simulink model "Lab3_12082026"  (R2019a)
settings: Solver=VariableStepAuto  StartTime=0.0  StopTime=10  RelTol=1e-3  EnableMultiTasking=on
libraries: dspsrcs4 x1, simulink x1
settings Model: Creator=CSE  LastModifiedBy=Admin
settings DataIOCC: ReturnWorkspaceOutputs=off
settings OptimizationCC: LifeSpan=inf
settings DebuggingCC: SFUnexpectedBacktrackingDiag=warning  SFNoUnconditionalDefaultTransitionDiag=warning  ArithmeticOperatorsInVariantConditions=warning
settings SFSimCC: SimUseLocalCustomCode=off
settings RTWCC: RTWUseLocalCustomCode=off
settings CodeAppCC: StateflowObjectComments=on
settings GRTTargetCC: TargetLangStandard=C89/C90 (ANSI)  GeneratePreprocessorConditionals=Disable all
settings ConfigComp: CovMetricSettings=dw  CovHtmlReporting=on  CovSaveCumulativeToWorkspaceVar=on  CovSaveSingleToWorkspaceVar=on  CovExternalEMLEnable=off

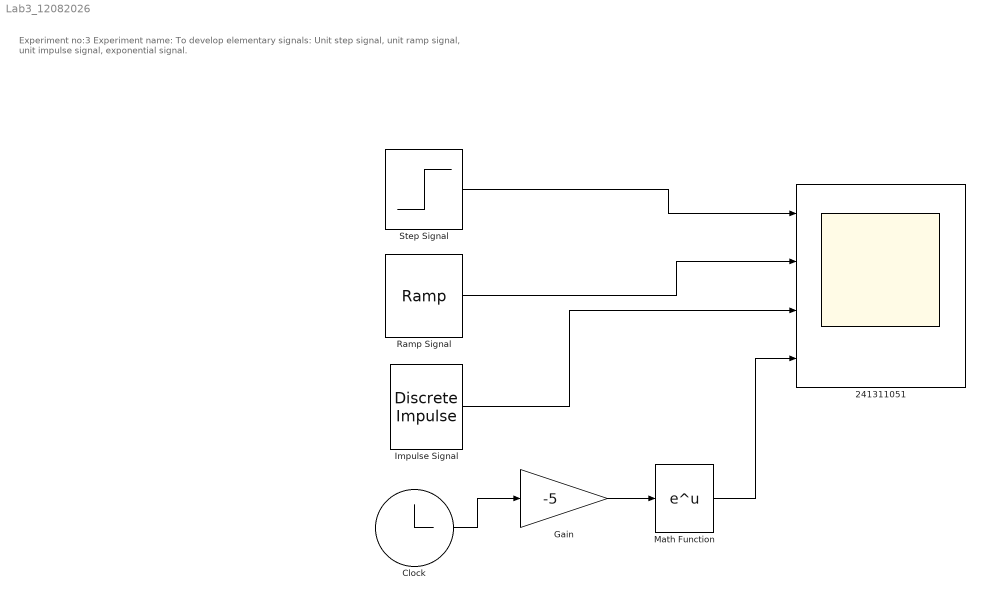
== system Lab3_12082026 ==
  note: Experiment no:3
      | Experiment name: To develop elementary signals: Unit step signal, unit ramp signal, unit impulse signal, exponential signal.
  241311051 : Scope  NumInputPorts=4
  "Clock " : Clock
  "Gain " : Gain  Gain=-5
  Impulse Signal : dspsrcs4/Discrete  Impulse  Delay=3  SampleTime=1  FrameSample=1  OutputFrames=off  dataType=double  isSigned=on  wordLen=16  udDataType=sfix(16)  fracBitsMode=Best precision  numFracBits=15  OutDataTypeStr=double  LastOutDataTypeStr=double
  "Math Function " : Math  SaturateOnIntegerOverflow=on
  Ramp Signal : simulink/Sources/Ramp  slope=2  start=0  InitialOutput=0
  Step Signal : Step  Time=2  SampleTime=0
  wires:
  Step Signal/1 -> 241311051/1
  Ramp Signal/1 -> 241311051/2
  Impulse Signal/1 -> 241311051/3
  "Clock "/1 -> "Gain "/1
  "Gain "/1 -> "Math Function "/1
  "Math Function "/1 -> 241311051/4
